simulink model "IMM_SVSF_VBL"  (R2020b)
settings: Solver=VariableStepAuto  StartTime=0  StopTime=imm_svsf.data.t(end)  FixedStep=.1  RelTol=1e-3
values from neighbouring files (symbols this model uses):
  A1 = [-2092.5 9351.9 -17282 16961 -9387.9 2860.7 -492.24 136.88 -72.802 20.041 1.6105]    [IMM_SVSF_VBL_init.m]
  A2 = [67006.6412715162	-355951.237408991	830816.525021041	-1120201.57641690	964579.013854285	-553286.067441687	213743.979431011	-54830.4962158105	8927.77493524045	-832.058541135094	37.1987933639492]    [IMM_SVSF_VBL_init.m]
  A3 = [7867.61770046033,-52053.6516069609,148124.836069431,-239805.009792072,245253.317990107,-165834.200826406,75160.6883321978,-22563.9811919106,4296.71317091153,-468.314195927266,25.6920380353340]    [IMM_SVSF_VBL_init.m]
  alpha = 0.5    [IMM_SVSF_VBL_init.m]
  bias = 0    [IMM_SVSF_VBL_init.m]
  delta = 0.1    [IMM_SVSF_VBL_init.m]
  Gamma = .38    (= 0.38)    [IMM_SVSF_VBL_init.m]
  P = diag([1e1,1e1,1e1,1e1,1e1,1e1])    [IMM_SVSF_VBL_init.m]
  Psi = 3.2    [IMM_SVSF_VBL_init.m]
  Q = diag([1e-8,1e-8,1e-8,1e-10,1e-10,1e-10])    [IMM_SVSF_VBL_init.m]
  R = [.5e-2 0;0  9.5e-2]    [IMM_SVSF_VBL_init.m]
  Wsoh = [1, .9 ,.8]    [IMM_SVSF_VBL_init.m]
  x0 = [0; 0;0;.85;0;0.01]    [IMM_SVSF_VBL_init.m]
undefined symbols (not defined in the file or in its folder): imm_svsf
settings Model: PauseTimes=10  OrderedModelArguments=off  Creator=Sara  LastModifiedBy=Sara
settings DataIOCC: SignalLogging=off  DSMLogging=off  ReturnWorkspaceOutputs=off

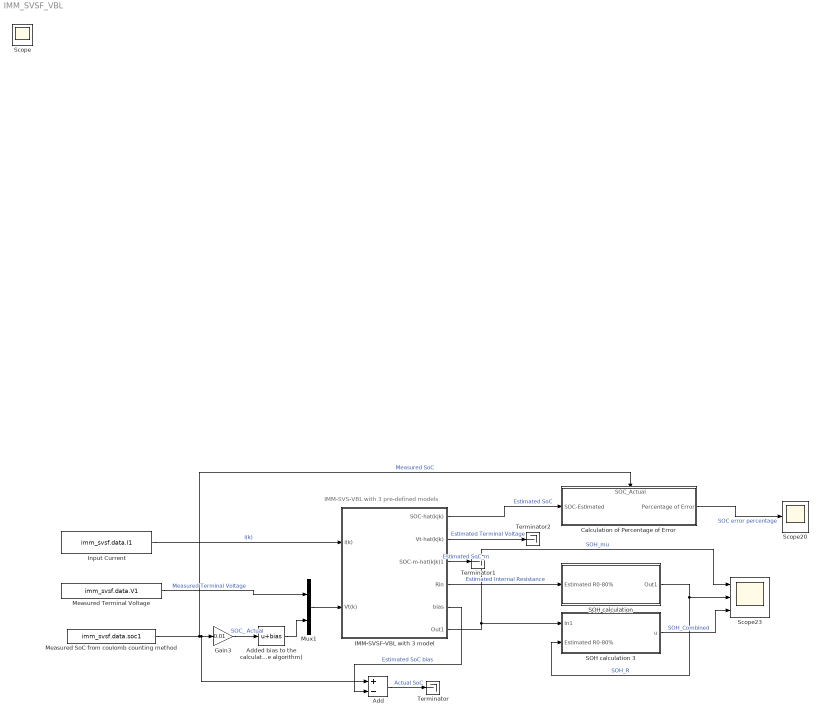
== system IMM_SVSF_VBL ==
  note: IMM-SVS-VBL with 3 pre-defined models
  Add : Sum  Inputs=+-
  Added bias to the calculated SoC (to test the algorithm) : Bias  Bias=bias
  Calculation of Percentage of Error : Subsystem
      settings: PortSchema="{\"entries\":[{\"content\":{\"sides\":[{\"content\":{\"connectorIds\":[\"In1\"]},\"type\":\"ConnectorPlacement.EquallySpacedRectSide\",\"uuid\":\"eac2cd31-9fdc-4543-87ad-aa5864e2159d\"},{\"content\":{\"connectorIds\":[\"Out1\"],\"side\":\"RIGHT\"},\"type\":\"ConnectorPlacement.EquallySpacedRectSide\",\"uuid\":\"1ecd87b5-9893-4496-a8be-b4dd1af22632\"},{\"content\":{\"connectorIds\":[\"In2\"],\"side\":\"TOP\"},\"type\":\"ConnectorPlacement.EquallySpacedRectSide\",\"uuid\":\"cd87a162-a144-48e6-b2b1-fbe5895e9416\"},{\"content\":{\"connectorIds\":[],\"side\":\"HIDDEN\"},\"type\":\"ConnectorPlacement.EquallySpacedRectSide\",\"uuid\":\"8217f259-f735-4e37-b118-d9f7cbe8fcbd\"}]},\"type\":\"ConnectorPlacement.EquallySpacedConnector\",\"uuid\":\"4f961f36-768e-4a3d-86d4-973ab0be26e4\"}],\"packageUris\":[\"http://schema.mathworks.com/mf0/Connector/R2020b\"],\"version\":\"1.0\"}"
  Gain3 : Gain  Gain=0.01
  IMM-SVSF-VBL with 3 model : Subsystem  mask{Eta=1, A=A1, DeltaT=delta, xhat_init=x0, Psi=Psi, Gamma=Gamma, R=R, P_init=P, transprob=[0.998 .001 0.001;.001 .998 0.001;0.001 0.001 .998], modeprob=[1/3;1/3;1/3]}
      mask prompts: Eta "Cell Coulombic efficiency, Eta"; A "Enter the OCV coefficients in a vector form as: [a10 a9 a8 a7 a6 a5 a4 a3 a2 a1 a0]"; DeltaT "Sampling time (Sec)"; xhat_init "Initial state estimation vector"; Psi "Saturation upper bound (Psi)"; R "Matrix R ( measurement noise covariance)"; P_init "Matrix P0"
      mask DialogControl DescGroupVar Prompt: Smooth variable structure filter (SVSF)
      mask DialogControl Control8 Prompt: Inputs (from up to down): 1-current, 2-terminal voltage
      mask DialogControl Control9 Prompt: Outputs (from up to down): 1-SOC estimate, 2-terminal voltage estimate
      mask DialogControl ParameterGroupVar Prompt: Phisical parameters of the Li-Ion cell:
      mask DialogControl Control6 Prompt: (Add text here)
      mask DialogControl Control5 Prompt: Simulation parameters:
  Input Current : FromWorkspace  VariableName=imm_svsf.data.I1  SampleTime=.1
  Measured SoC from coulomb counting method : FromWorkspace  VariableName=imm_svsf.data.soc1  SampleTime=.1
  Measured Terminal Voltage : FromWorkspace  VariableName=imm_svsf.data.V1  SampleTime=.1
  Mux1 : Mux  Inputs=2
  "SOH calculation " : Subsystem
  SOH calculation 3 : Subsystem
  Scope20 : Scope
  Scope23 : Scope  NumInputPorts=3
  Terminator : Terminator
  Terminator1 : Terminator
  Terminator2 : Terminator
  Scope : Scope
  wires:
  Measured Terminal Voltage/1 -> Mux1/1  "Measured Terminal Voltage"
  Mux1/1 -> IMM-SVSF-VBL with 3 model/2(Vt(k))
  Gain3/1 -> Added bias to the calculated SoC (to test the algorithm)/1  "SOC_ Actual"
  Input Current/1 -> IMM-SVSF-VBL with 3 model/1(i(k))  "i(k)"
  Added bias to the calculated SoC (to test the algorithm)/1 -> Mux1/2
  IMM-SVSF-VBL with 3 model/1(SOC-hat(k|k)) -> Calculation of Percentage of Error/1(SOC-Estimated)  "Estimated SoC"
  Measured SoC from coulomb counting method/1 -> Calculation of Percentage of Error/2(SOC_Actual), Add/1, Gain3/1  "Measured SoC"
  Calculation of Percentage of Error/1(Percentage of Error) -> Scope20/1  "SOC error percentage"
  "SOH calculation "/1(Out1) -> SOH calculation 3/2(Estimated R0-80%), Scope23/2  "SOH_R"
  SOH calculation 3/1(u) -> Scope23/3  "SOH_Combined"
  IMM-SVSF-VBL with 3 model/4(Rin) -> "SOH calculation "/1(Estimated R0-80%)  "Estimated Internal Resistance"
  IMM-SVSF-VBL with 3 model/6(Out1) -> Scope23/1, SOH calculation 3/1(In1)  "SOH_mu"
  IMM-SVSF-VBL with 3 model/5(bias) -> Add/2  "Estimated SoC bias"
  Add/1 -> Terminator/1  "Actual SoC"
  IMM-SVSF-VBL with 3 model/3(SOC-m-hat(k|k)1) -> Terminator1/1  "Estimated SoC_m"
  IMM-SVSF-VBL with 3 model/2(Vt-hat(k|k)) -> Terminator2/1  "Estimated Terminal Voltage"

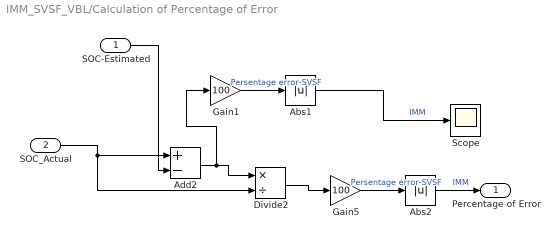
== system IMM_SVSF_VBL/Calculation of Percentage of Error ==
  SOC-Estimated : Inport
  SOC_Actual : Inport  Port=2
  Abs1 : Abs
  Abs2 : Abs
  Add2 : Sum  Inputs=+-
  Divide2 : Product  Inputs=*/
  Gain1 : Gain  Gain=100
  Gain5 : Gain  Gain=100
  Scope : Scope
  Percentage of Error : Outport
  wires:
  SOC_Actual/1 -> Divide2/2, Add2/1
  Gain5/1 -> Abs2/1  "Persentage error-SVSF"
  SOC-Estimated/1 -> Add2/2
  Divide2/1 -> Gain5/1
  Abs2/1 -> Percentage of Error/1  "IMM"
  Abs1/1 -> Scope/1  "IMM"
  Gain1/1 -> Abs1/1  "Persentage error-SVSF"
  Add2/1 -> Gain1/1, Divide2/1

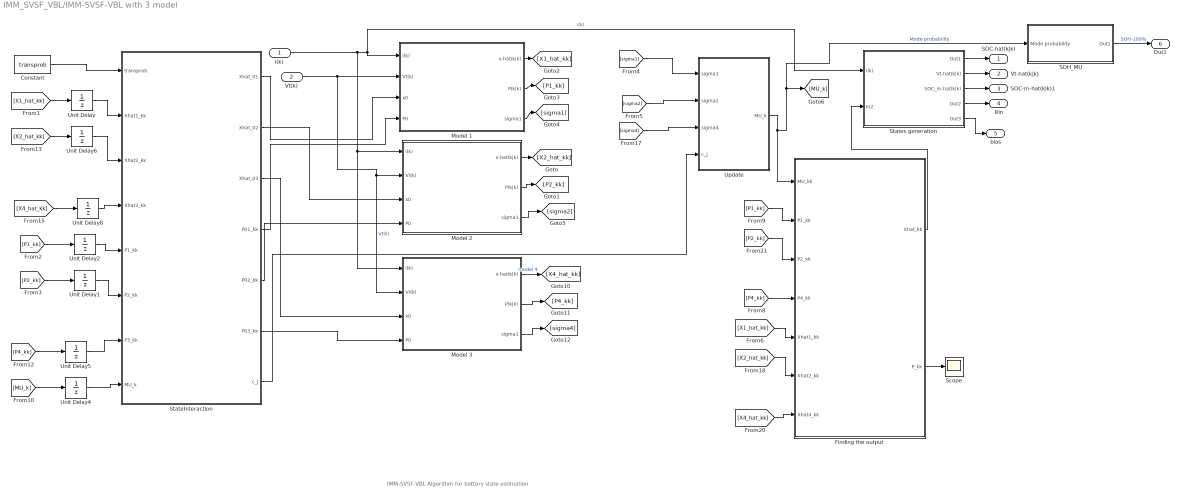
== system IMM_SVSF_VBL/IMM-SVSF-VBL with 3 model ==
  note: IMM-SVSF-VBL Algorithm for battery state estimation
  i(k) : Inport
  Vt(k) : Inport  Port=2
  Constant : Constant  Value=transprob  SampleTime=DeltaT
  Finding the output : MATLAB Function  TreatAsAtomicUnit=on
  Model 1 : Subsystem  mask{A=A1, Q=Q}
      mask prompts: A "Enter the OCV coefficients in a vector form as: [a10 a9 a8 a7 a6 a5 a4 a3 a2 a1 a0]"; Q "Covariance process noise"
      mask DialogControl DescGroupVar Prompt: Smooth variable structure filter (SVSF)
      mask DialogControl Control8 Prompt: Inputs (from up to down): 1-current, 2-terminal voltage
      mask DialogControl Control9 Prompt: Outputs (from up to down): 1-SOC estimate, 2-terminal voltage estimate
      mask DialogControl ParameterGroupVar Prompt: Phisical parameters of the Li-Ion cell:
      mask DialogControl Control6 Prompt: (Add text here)
      mask DialogControl Control5 Prompt: Simulation parameters:
  Model 2 : Subsystem  mask{A=A2, Q=Q}
      mask prompts: A "Enter the OCV coefficients in a vector form as: [a10 a9 a8 a7 a6 a5 a4 a3 a2 a1 a0]"; Q "Covariance process noise"
      mask DialogControl DescGroupVar Prompt: Smooth variable structure filter (SVSF)
      mask DialogControl Control8 Prompt: Inputs (from up to down): 1-current, 2-terminal voltage
      mask DialogControl Control9 Prompt: Outputs (from up to down): 1-SOC estimate, 2-terminal voltage estimate
      mask DialogControl ParameterGroupVar Prompt: Phisical parameters of the Li-Ion cell:
      mask DialogControl Control6 Prompt: (Add text here)
      mask DialogControl Control5 Prompt: Simulation parameters:
  Model 3 : Subsystem  mask{A=A3, Q=Q}
      mask prompts: A "Enter the OCV coefficients in a vector form as: [a10 a9 a8 a7 a6 a5 a4 a3 a2 a1 a0]"; Q "Covariance process noise"
      mask DialogControl DescGroupVar Prompt: Smooth variable structure filter (SVSF)
      mask DialogControl Control8 Prompt: Inputs (from up to down): 1-current, 2-terminal voltage
      mask DialogControl Control9 Prompt: Outputs (from up to down): 1-SOC estimate, 2-terminal voltage estimate
      mask DialogControl ParameterGroupVar Prompt: Phisical parameters of the Li-Ion cell:
      mask DialogControl Control6 Prompt: (Add text here)
      mask DialogControl Control5 Prompt: Simulation parameters:
  SOH_MU : Subsystem
  Scope : Scope
  StateInteraction : MATLAB Function  TreatAsAtomicUnit=on
  States generation : Subsystem
  Unit Delay : UnitDelay  InitialCondition=xhat_init  SampleTime=DeltaT  HasFrameUpgradeWarning=on
  Unit Delay1 : UnitDelay  InitialCondition=P_init  SampleTime=DeltaT  HasFrameUpgradeWarning=on
  Unit Delay2 : UnitDelay  InitialCondition=P_init  SampleTime=DeltaT  HasFrameUpgradeWarning=on
  Unit Delay4 : UnitDelay  InitialCondition=modeprob  SampleTime=DeltaT  HasFrameUpgradeWarning=on
  Unit Delay5 : UnitDelay  InitialCondition=P_init  SampleTime=DeltaT  HasFrameUpgradeWarning=on
  Unit Delay6 : UnitDelay  InitialCondition=xhat_init  SampleTime=DeltaT  HasFrameUpgradeWarning=on
  Unit Delay8 : UnitDelay  InitialCondition=xhat_init  SampleTime=DeltaT  HasFrameUpgradeWarning=on
  Update : MATLAB Function  TreatAsAtomicUnit=on
  SOC-hat(k|k) : Outport  VectorParamsAs1DForOutWhenUnconnected=off
  Vt-hat(k|k) : Outport  Port=2  VectorParamsAs1DForOutWhenUnconnected=off
  SOC-m-hat(k|k)1 : Outport  Port=3  VectorParamsAs1DForOutWhenUnconnected=off
  Rin : Outport  Port=4  VectorParamsAs1DForOutWhenUnconnected=off
  bias : Outport  Port=5  VectorParamsAs1DForOutWhenUnconnected=off
  Out1 : Outport  Port=6
  wires:
  Unit Delay/1 -> StateInteraction/2(Xhat1_kk)
  Model 2/2(P(k|k)) -> [P2_kk]
  Model 1/2(P(k|k)) -> [P1_kk]
  Unit Delay2/1 -> StateInteraction/5(P1_kk)
  Model 1/3(sigma1) -> [sigma1]
  Model 2/3(sigma1) -> [sigma2]
  [P1_kk] -> Finding the output/2(P1_kk)
  [MU_k] -> Unit Delay4/1
  Unit Delay4/1 -> StateInteraction/8(MU_k)
  Finding the output/2(P_kk) -> Scope/1
  i(k)/1 -> Model 2/1(i(k)), Model 3/1(i(k)), Model 1/1(i(k)), States generation/1(i(k))  "i(k)"
  Model 3/3(sigma1) -> [sigma4]
  Vt(k)/1 -> Model 1/2(Vt(k)), Model 2/2(Vt(k)), Model 3/2(Vt(k))  "Vt(k)"
  Model 3/2(P(k|k)) -> [P4_kk]
  StateInteraction/6(P03_kk) -> Model 3/4(P0)
  StateInteraction/2(Xhat_02) -> Model 2/3(x0)
  StateInteraction/1(Xhat_01) -> Model 1/3(x0)
  StateInteraction/4(P01_kk) -> Model 1/4(P0)
  StateInteraction/5(P02_kk) -> Model 2/4(P0)
  StateInteraction/3(Xhat_03) -> Model 3/3(x0)
  [P1_kk] -> Unit Delay2/1
  [P4_kk] -> Unit Delay5/1
  [P2_kk] -> Unit Delay1/1
  [X1_hat_kk] -> Unit Delay/1
  [X4_hat_kk] -> Unit Delay8/1
  [X2_hat_kk] -> Unit Delay6/1
  [sigma4] -> Update/3(sigma4)
  [sigma2] -> Update/2(sigma2)
  [sigma1] -> Update/1(sigma1)
  [X1_hat_kk] -> Finding the output/5(Xhat1_kk)
  [X4_hat_kk] -> Finding the output/7(Xhat4_kk)
  [X2_hat_kk] -> Finding the output/6(Xhat2_kk)
  [P2_kk] -> Finding the output/3(P2_kk)
  [P4_kk] -> Finding the output/4(P4_kk)
  Unit Delay1/1 -> StateInteraction/6(P2_kk)
  Unit Delay5/1 -> StateInteraction/7(P3_kk)
  Unit Delay6/1 -> StateInteraction/3(Xhat2_kk)
  Unit Delay8/1 -> StateInteraction/4(Xhat3_kk)
  Constant/1 -> StateInteraction/1(transprob)
  Finding the output/1(Xhat_kk) -> States generation/2(In2)
  States generation/1(Out1) -> SOC-hat(k|k)/1
  States generation/2(Vt-hat(k|k)) -> Vt-hat(k|k)/1
  Model 2/1(x-hat(k|k)) -> [X2_hat_kk]
  Model 1/1(x-hat(k|k)) -> [X1_hat_kk]
  States generation/3(SOC_m-hat(k|k)) -> SOC-m-hat(k|k)1/1
  States generation/4(Out2) -> Rin/1
  States generation/5(Out3) -> bias/1
  StateInteraction/7(c_j) -> Update/4(c_j)
  SOH_MU/1(Out1) -> Out1/1  "SOH-100%"
  Update/1(MU_k) -> SOH_MU/1(Mode probability), [MU_k], Finding the output/1(MU_kk)  "Mode probability"
  Model 3/1(x-hat(k|k)) -> [X4_hat_kk]  "model 4"

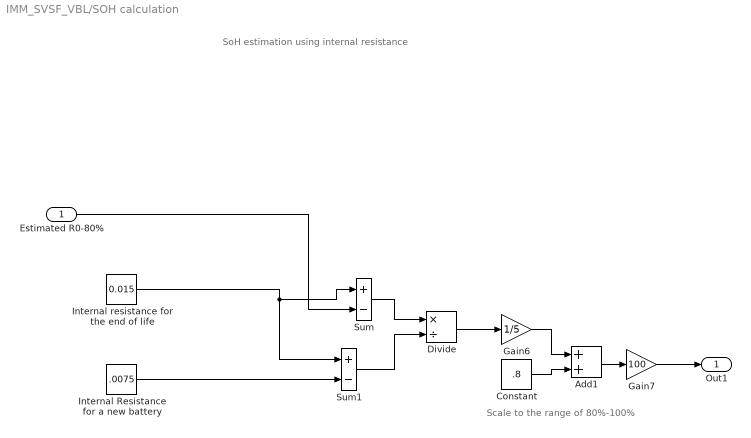
== system IMM_SVSF_VBL/SOH calculation  ==
  note: Scale to the range of 80%-100%
  note: SoH estimation using internal resistance
  Estimated R0-80% : Inport
  Add1 : Sum
  Constant : Constant  Value=.8
  Divide : Product  Inputs=*/
  Gain6 : Gain  Gain=1/5
  Gain7 : Gain  Gain=100
  "Internal Resistance for a new battery " : Constant  Value=.0075
  "Internal resistance for the end of life " : Constant  Value=0.015
  Sum : Sum  Inputs=+-
  Sum1 : Sum  Inputs=+-
  Out1 : Outport
  wires:
  "Internal resistance for the end of life "/1 -> Sum1/1, Sum/1
  "Internal Resistance for a new battery "/1 -> Sum1/2
  Gain6/1 -> Add1/1
  Constant/1 -> Add1/2
  Divide/1 -> Gain6/1
  Sum1/1 -> Divide/2
  Sum/1 -> Divide/1
  Add1/1 -> Gain7/1
  Gain7/1 -> Out1/1
  Estimated R0-80%/1 -> Sum/2

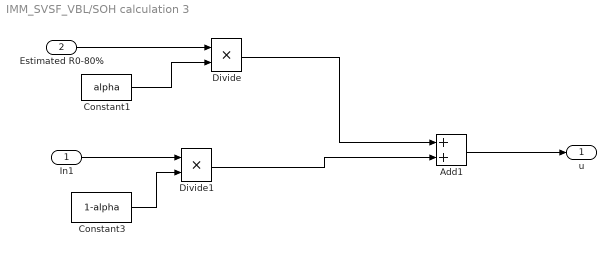
== system IMM_SVSF_VBL/SOH calculation 3 ==
  In1 : Inport
  Estimated R0-80% : Inport  Port=2
  Add1 : Sum
  Constant1 : Constant  Value=alpha
  Constant3 : Constant  Value=1-alpha
  Divide : Product  Inputs=**
  Divide1 : Product  Inputs=**
  u : Outport
  wires:
  Constant1/1 -> Divide/2
  Estimated R0-80%/1 -> Divide/1
  Add1/1 -> u/1
  In1/1 -> Divide1/1
  Constant3/1 -> Divide1/2
  Divide/1 -> Add1/1
  Divide1/1 -> Add1/2

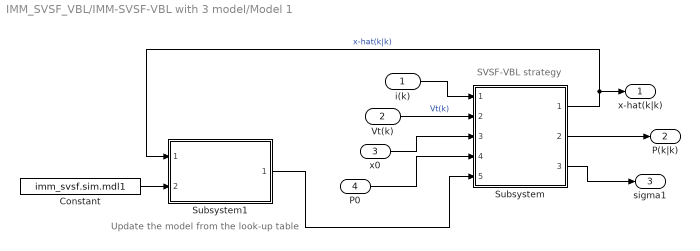
== system IMM_SVSF_VBL/IMM-SVSF-VBL with 3 model/Model 1 ==
  note: SVSF-VBL strategy
  note: Update the model from the look-up table
  i(k) : Inport
  Vt(k) : Inport  Port=2
  x0 : Inport  Port=3
  P0 : Inport  Port=4
  Constant : Constant  Value=imm_svsf.sim.mdl1
  Subsystem : Subsystem  ReferencedSubsystem=XinSVSF3rd
  Subsystem1 : Subsystem  ReferencedSubsystem=parmeter_lookup_svsf
  x-hat(k|k) : Outport  VectorParamsAs1DForOutWhenUnconnected=off
  P(k|k) : Outport  Port=2
  sigma1 : Outport  Port=3
  wires:
  i(k)/1 -> Subsystem/1
  Vt(k)/1 -> Subsystem/2  "Vt(k)"
  x0/1 -> Subsystem/3
  P0/1 -> Subsystem/4
  Subsystem/2 -> P(k|k)/1
  Subsystem/3 -> sigma1/1
  Subsystem/1 -> Subsystem1/1, x-hat(k|k)/1  "x-hat(k|k)"
  Constant/1 -> Subsystem1/2
  Subsystem1/1 -> Subsystem/5

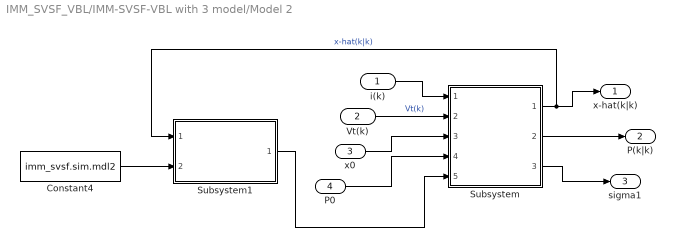
== system IMM_SVSF_VBL/IMM-SVSF-VBL with 3 model/Model 2 ==
  i(k) : Inport
  Vt(k) : Inport  Port=2
  x0 : Inport  Port=3
  P0 : Inport  Port=4
  Constant4 : Constant  Value=imm_svsf.sim.mdl2
  Subsystem : Subsystem  ReferencedSubsystem=XinSVSF3rd
  Subsystem1 : Subsystem  ReferencedSubsystem=parmeter_lookup_svsf
  x-hat(k|k) : Outport  VectorParamsAs1DForOutWhenUnconnected=off
  P(k|k) : Outport  Port=2
  sigma1 : Outport  Port=3
  wires:
  Subsystem/3 -> sigma1/1
  x0/1 -> Subsystem/3
  Subsystem/2 -> P(k|k)/1
  P0/1 -> Subsystem/4
  i(k)/1 -> Subsystem/1
  Vt(k)/1 -> Subsystem/2  "Vt(k)"
  Subsystem/1 -> Subsystem1/1, x-hat(k|k)/1  "x-hat(k|k)"
  Constant4/1 -> Subsystem1/2
  Subsystem1/1 -> Subsystem/5

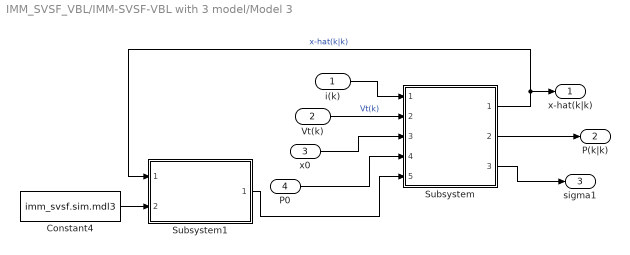
== system IMM_SVSF_VBL/IMM-SVSF-VBL with 3 model/Model 3 ==
  i(k) : Inport
  Vt(k) : Inport  Port=2
  x0 : Inport  Port=3
  P0 : Inport  Port=4
  Constant4 : Constant  Value=imm_svsf.sim.mdl3
  Subsystem : Subsystem  ReferencedSubsystem=XinSVSF3rd
  Subsystem1 : Subsystem  ReferencedSubsystem=parmeter_lookup_svsf
  x-hat(k|k) : Outport  VectorParamsAs1DForOutWhenUnconnected=off
  P(k|k) : Outport  Port=2
  sigma1 : Outport  Port=3
  wires:
  Vt(k)/1 -> Subsystem/2  "Vt(k)"
  i(k)/1 -> Subsystem/1
  P0/1 -> Subsystem/4
  x0/1 -> Subsystem/3
  Subsystem/3 -> sigma1/1
  Subsystem/2 -> P(k|k)/1
  Subsystem/1 -> Subsystem1/1, x-hat(k|k)/1  "x-hat(k|k)"
  Constant4/1 -> Subsystem1/2
  Subsystem1/1 -> Subsystem/5

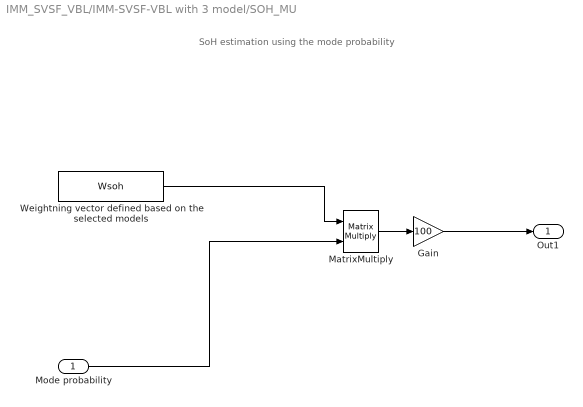
== system IMM_SVSF_VBL/IMM-SVSF-VBL with 3 model/SOH_MU ==
  note: SoH estimation using the mode probability
  Mode probability : Inport
  Gain : Gain  Gain=100
  MatrixMultiply : Product  Multiplication=Matrix(*)
  "Weightning vector defined based on the selected models " : Constant  Value=Wsoh  VectorParams1D=off
  Out1 : Outport
  wires:
  "Weightning vector defined based on the selected models "/1 -> MatrixMultiply/1
  Mode probability/1 -> MatrixMultiply/2
  MatrixMultiply/1 -> Gain/1
  Gain/1 -> Out1/1

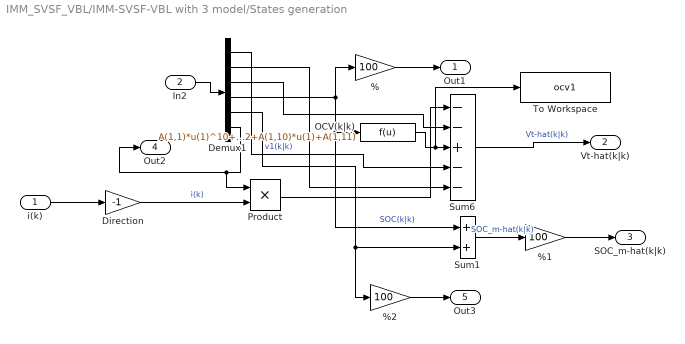
== system IMM_SVSF_VBL/IMM-SVSF-VBL with 3 model/States generation ==
  i(k) : Inport
  In2 : Inport  Port=2
  % : Gain  Gain=100  SampleTime=DeltaT
  %1 : Gain  Gain=100  SampleTime=DeltaT
  %2 : Gain  Gain=100  SampleTime=DeltaT
  Demux1 : Demux  Outputs=6
  Direction : Gain  Gain=-1  SampleTime=DeltaT
  OCV(k|k) : Fcn  Expr=A(1,1)*u(1)^10+A(1,2)*u(1)^9+A(1,3)*u(1)^8+A(1,4)*u(1)^7+A(1,5)*u(1)^6+A(1,6)*u(1)^5+A(1,7)*u(1)^4+A(1,8)*u(1)^3+A(1,9)*u(1)^2+A(1,10)*u(1)+A(1,11)  SampleTime=DeltaT
  Product : Product
  Sum1 : Sum  SampleTime=DeltaT
  Sum6 : Sum  Inputs=--+--  SampleTime=DeltaT
  To Workspace : ToWorkspace  VariableName=ocv1  SaveFormat=Structure With Time  SampleTime=-1
  Out1 : Outport
  Vt-hat(k|k) : Outport  Port=2
  SOC_m-hat(k|k) : Outport  Port=3
  Out2 : Outport  Port=4
  Out3 : Outport  Port=5
  wires:
  Product/1 -> Sum6/1
  i(k)/1 -> Direction/1
  Demux1/4 -> %/1, OCV(k|k)/1, Sum1/1  "SOC(k|k)"
  Demux1/1 -> Sum6/4  "v1(k|k)"
  Sum6/1 -> Vt-hat(k|k)/1  "Vt-hat(k|k)"
  OCV(k|k)/1 -> To Workspace/1, Sum6/3
  Direction/1 -> Product/2  "i(k)"
  In2/1 -> Demux1/1
  %/1 -> Out1/1
  Demux1/2 -> Sum6/5
  Demux1/6 -> Out2/1, Product/1
  Demux1/5 -> %2/1, Sum1/2
  Sum1/1 -> %1/1  "SOC_m-hat(k|k)"
  %1/1 -> SOC_m-hat(k|k)/1
  %2/1 -> Out3/1
  Demux1/3 -> Sum6/2

== matlab function IMM_SVSF_VBL/IMM-SVSF-VBL with 3 model/Finding the output ==
  data: MU_kk input; P1_kk input; P2_kk input; P4_kk input; Xhat1_kk input; Xhat_kk output; P_kk output; Xhat2_kk input; Xhat4_kk input
function [Xhat_kk,P_kk]  = StateEstimate(MU_kk,P1_kk,P2_kk, P4_kk, Xhat1_kk, Xhat2_kk,Xhat4_kk)
% This step is for finding the output and it doesn't change any part of the
% algorithm
%Estimation and covariance combination 

Xhat_kk = Xhat1_kk* MU_kk(1) + Xhat2_kk* MU_kk(2) + ...
    Xhat4_kk* MU_kk(3); %equation 11.6.6-17



P_kk = MU_kk(1)*(P1_kk + (Xhat1_kk - Xhat_kk)*(Xhat1_kk-Xhat_kk)')+...
       MU_kk(2)*(P2_kk + (Xhat2_kk -Xhat_kk)*(Xhat2_kk -Xhat_kk)')+...
       MU_kk(3)*(P4_kk + (Xhat4_kk-Xhat_kk)*(Xhat4_kk-Xhat_kk)');
%        MU_kk(4)*(P4_kk + (Xhat4_kk-Xhat_kk)*(Xhat4_kk-Xhat_kk)'); % equation 11.6.6-18

% P_kk = .01*ones(2,2);


end

== matlab function IMM_SVSF_VBL/IMM-SVSF-VBL with 3 model/StateInteraction ==
  data: transprob input; Xhat_01 output; Xhat_02 output; Xhat_03 output; Xhat1_kk input; Xhat2_kk input; Xhat3_kk input; P1_kk input; P2_kk input; P3_kk input; P01_kk output; MU_k input; P02_kk output; P03_kk output; c_j output
function [Xhat_01,Xhat_02,Xhat_03, P01_kk, P02_kk,P03_kk,c_j] = StateInteraction(transprob, Xhat1_kk,Xhat2_kk,Xhat3_kk, P1_kk,P2_kk, P3_kk, MU_k)

 r = 3;
 MU_kk = zeros(3,3);

% Mixing probabilities calculation
c_j = transprob'*MU_k; % (rxr)' * (rx1)   equation 11.6.6-8
%STEP 1

for j = 1:r
            for i = 1:r
                % caluclate mixing probabilities equation 11.6.6-7 
                MU_kk(i,j) = (1/c_j(j))*transprob(i,j)*MU_k(i);
            end
end

% Mixed initial states and Covariances 
%STEP 2
Xhat_01 = Xhat1_kk* MU_kk(1,1)+ Xhat2_kk* MU_kk(2,1)+Xhat3_kk* MU_kk(3,1);% mixing initial state, equation 11.6.6-9
Xhat_02 = Xhat1_kk* MU_kk(1,2)+ Xhat2_kk* MU_kk(2,2)+Xhat3_kk* MU_kk(3,2);% mixing initial state, equation 11.6.6-9
Xhat_03 = Xhat1_kk* MU_kk(1,3)+ Xhat2_kk* MU_kk(2,3)+Xhat3_kk* MU_kk(3,3);% mixing initial state, equation 11.6.6-9

%STEP3
P01_kk = MU_kk(1,1)*(P1_kk + (Xhat1_kk - Xhat_01)*(Xhat1_kk - Xhat_01)')+...
    MU_kk(2,1)*(P2_kk+ (Xhat2_kk- Xhat_02)*(Xhat2_kk - Xhat_02)')+...
    MU_kk(3,1)*(P3_kk + (Xhat3_kk - Xhat_03)*(Xhat3_kk - Xhat_03)');% mixing initial covariance, equation 11.6.6-10

P02_kk = MU_kk(1,2)*(P1_kk + (Xhat1_kk - Xhat_01)*(Xhat1_kk - Xhat_01)')+...
    MU_kk(2,2)*(P2_kk+ (Xhat2_kk - Xhat_02)*(Xhat2_kk - Xhat_02)')+...
    MU_kk(3,2)*(P3_kk + (Xhat3_kk - Xhat_03)*(Xhat3_kk - Xhat_03)');% mixing initial covariance,equation 11.6.6-10

P03_kk = MU_kk(1,3)*(P1_kk + (Xhat1_kk - Xhat_01)*(Xhat1_kk - Xhat_01)')+...
    MU_kk(2,3)*(P2_kk+ (Xhat2_kk - Xhat_02)*(Xhat2_kk - Xhat_02)')+...
    MU_kk(3,3)*(P3_kk + (Xhat3_kk - Xhat_03)*(Xhat3_kk - Xhat_03)');% mixing initial covariance,equation 11.6.6-10

end

== matlab function IMM_SVSF_VBL/IMM-SVSF-VBL with 3 model/Update ==
  data: sigma1 input; sigma2 input; sigma4 input; MU_k output; c_j input
function MU_k   = update(sigma1,sigma2,sigma4, c_j)



%%
%    cj_bar = zeros([4,1]);    
%     
%     for j = 1:4
%         c_j = 0;
%         for i = 1:4
%             c_j = c_j + transprob(i,j)*MU_k_1(i);
%         end
%         
%         cj_bar(j) = c_j;
%         
%     end
%c_j = transprob'*MU_k_1;
%MU_kk = transprob.*(MU_k_1*(1/c_j));
%%

cbar1 = c_j(1,:);
cbar2 = c_j(2,:);
% cbar3 = c_j(3,:);
cbar4 = c_j(3,:);

sigma1 = sigma1;
sigma2 = sigma2;
% sigma3 = sigma3;
sigma4 = sigma4;

c= sigma1*cbar1 + sigma2*cbar2 + sigma4*cbar4;

MU_k1 = (1/c)* sigma1 * cbar1;
MU_k2 = (1/c)* sigma2 * cbar2;
MU_k4 = (1/c)* sigma4 * cbar4;
% MU_k4 = (1/c)* sigma4 * cbar4;

MU_k =[MU_k1;MU_k2;MU_k4];



end
